simulink model "ADC_Model"  (R2016a)
settings: Solver=ode4  StartTime=t0  StopTime=tf  FixedStep=dt  RelTol=1e-6
InitFcn:
  | sat_model_init
values from neighbouring files (symbols this model uses):
  bias0 = 3/3600*randn(3,1)*pi/180    [sat_model_init.m]
  epoch = [2017 06 01 00 00 00]    [sat_model_init.m]
  gyro_freq = 25    [sat_model_init.m]
  I_max = 1.0    (= 1)    [sat_model_init.m]
  J = [1 ... (first row only)    [sat_model_init.m]
  J_c = [Jx  0  0 ... (first row only)    [sat_model_init.m]
  m = 9    [sat_model_init.m]
  mag_freq = 10    [sat_model_init.m]
  mu = 3.986004415e14    (= 398600441500000)    [sat_model_init.m]
  q0 = [1 ... (first row only)    [sat_model_init.m]
  r0 = (ROT3(omega)*ROT1(inc)*ROT3(Omega))'*[r0*cos(f0) ... (first row only)    [sat_model_init.m]
  Re = 6378.1363e3    (= 6378136.3)    [sat_model_init.m]
  sig_B = 4.5e-8    (= 4.5e-08)    [sat_model_init.m]
  sig_s = 0.1    [sat_model_init.m]
  sig_u = 1*pi/180*1/3600    (= 4.8481368111e-06)    [sat_model_init.m]
  sig_v = (0.0066*pi/180)*2    (= 0.000230383461263)    [sat_model_init.m]
  SP = 4.57e-5    (= 4.57e-05)    [sat_model_init.m]
  sun_freq = 10    [sat_model_init.m]
  v0 = (ROT3(omega)*ROT1(inc)*ROT3(Omega))'*[-mu/h*sin(f0) ... (first row only)    [sat_model_init.m]
  w0 = 0.2*ones(3,1)/sqrt(3)    [sat_model_init.m]
  w_earth = 7.2921158553e-5    (= 7.2921158553e-05)    [sat_model_init.m]
undefined symbols (not defined in the file or in its folder): FACET_model
libraries: vrlib x4
settings Model: Creator=Josue  LastModifiedBy=Graham Voysey
settings DataIOCC: LimitDataPoints=on  SaveFormat=Array  SignalLoggingSaveFormat=ModelDataLogs  SaveState=on
settings OptimizationCC: ExpressionDepthLimit=2147483647  EfficientMapNaN2IntZero=off
settings DebuggingCC: ReadBeforeWriteMsg=DisableAll  WriteAfterWriteMsg=DisableAll  WriteAfterReadMsg=DisableAll  UnderspecifiedInitializationDetection=Classic  MergeDetectMultiDrivingBlocksExec=none  SolverPrmCheckMsg=warning  MultiTaskDSMMsg=warning  MultiTaskCondExecSysMsg=none  FcnCallInpInsideContextMsg=UseLocalSettings  StateNameClashWarn=warning
settings HardwareCC: ProdBitPerPointer=32  ProdLargestAtomicFloat=None  ProdIntDivRoundTo=Undefined  ProdEndianess=Unspecified  ProdWordSize=32  ProdHWDeviceType=32-bit Generic  TargetBitPerPointer=64  TargetLongLongMode=on  TargetIntDivRoundTo=Zero  TargetEndianess=LittleEndian  TargetWordSize=64  TargetHWDeviceType=MATLAB Host  ProdEqTarget=off
settings ModelReferenceCC: PropagateSignalLabelsOutOfModel=off
settings SFSimCC: SimParseCustomCode=off
settings CodeAppCC: MaxIdLength=128
settings GRTTargetCC: CombineOutputUpdateFcns=off  GRTInterface=on
settings ConfigComp: CovModelRefEnable=Off

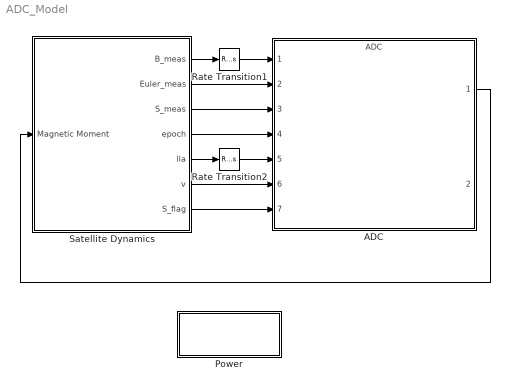
== system ADC_Model ==
  ADC : ModelReference  ModelNameDialog=ADC  SimulationMode=Normal  ModelReferenceVersion=1.1171
  Power : Subsystem
  Rate Transition1 : RateTransition  OutPortSampleTime=.1
  Rate Transition2 : RateTransition  OutPortSampleTime=.1
  Satellite Dynamics : Subsystem
  wires:
  Satellite Dynamics/4(epoch) -> ADC/4
  Satellite Dynamics/1(B_meas) -> Rate Transition1/1
  Satellite Dynamics/2(Euler_meas) -> ADC/2
  Satellite Dynamics/3(S_meas) -> ADC/3
  Satellite Dynamics/5(lla) -> Rate Transition2/1
  Satellite Dynamics/7(S_flag) -> ADC/7
  ADC/1 -> Satellite Dynamics/1(Magnetic Moment)
  Satellite Dynamics/6(v) -> ADC/6
  Rate Transition1/1 -> ADC/1
  Rate Transition2/1 -> ADC/5

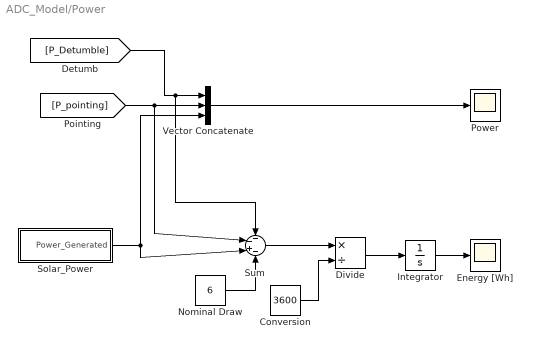
== system ADC_Model/Power ==
  Conversion : Constant  Value=3600
  Divide : Product  Inputs=*/
  Energy [Wh] : Scope
  Integrator : Integrator  InitialCondition=25  LimitOutput=on  UpperSaturationLimit=30  LowerSaturationLimit=0
  Nominal Draw : Constant  Value=6
  Power : Scope
  Solar_Power : Subsystem
  Sum : Sum  Inputs=--+-
  Vector Concatenate : Concatenate  NumInputs=3
  wires:
  [P_Detumble] -> Vector Concatenate/1, Sum/1
  Vector Concatenate/1 -> Power/1
  [P_pointing] -> Sum/2, Vector Concatenate/2
  Solar_Power/1(Power_Generated) -> Vector Concatenate/3, Sum/3
  Nominal Draw/1 -> Sum/4
  Integrator/1 -> Energy [Wh]/1
  Divide/1 -> Integrator/1
  Conversion/1 -> Divide/2
  Sum/1 -> Divide/1

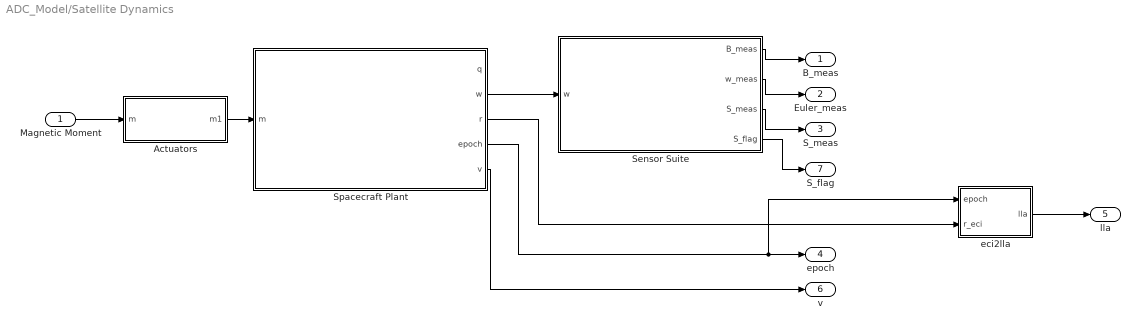
== system ADC_Model/Satellite Dynamics ==
  Magnetic Moment : Inport
  Actuators : Subsystem
  Sensor Suite : Subsystem
  Spacecraft Plant : Subsystem
  eci2lla : MATLAB Function  TreatAsAtomicUnit=on
  B_meas : Outport
  Euler_meas : Outport  Port=2
  S_meas : Outport  Port=3
  epoch : Outport  Port=4
  lla : Outport  Port=5
  v : Outport  Port=6
  S_flag : Outport  Port=7
  wires:
  Spacecraft Plant/2(w) -> Sensor Suite/1(w)
  Magnetic Moment/1 -> Actuators/1(m)
  Sensor Suite/1(B_meas) -> B_meas/1
  Sensor Suite/2(w_meas) -> Euler_meas/1
  Sensor Suite/3(S_meas) -> S_meas/1
  Actuators/1(m1) -> Spacecraft Plant/1(m)
  Spacecraft Plant/5(v) -> v/1
  Spacecraft Plant/4(epoch) -> eci2lla/1(epoch), epoch/1
  Sensor Suite/4(S_flag) -> S_flag/1
  eci2lla/1(lla) -> lla/1
  Spacecraft Plant/3(r) -> eci2lla/2(r_eci)

== system ADC_Model/Power/Solar_Power ==
  Constant2 : Constant  Value=Re
  Constant3 : Constant  Value=FACET_model.Asolar
  Constant6 : Constant  Value=FACET_model.n
  Constant8 : Constant  Value=FACET_model.num_of_faces
  Embedded MATLAB Function : MATLAB Function  TreatAsAtomicUnit=on
  Power_Generated : Outport
  wires:
  Embedded MATLAB Function/1(Power) -> Power_Generated/1
  [R_BtoECI] -> Embedded MATLAB Function/6(R_BtoECI)
  [R_SUN] -> Embedded MATLAB Function/1(R_SUN)
  Constant8/1 -> Embedded MATLAB Function/4(faces)
  [r] -> Embedded MATLAB Function/2(r)
  Constant6/1 -> Embedded MATLAB Function/3(n)
  Constant2/1 -> Embedded MATLAB Function/5(Re)
  Constant3/1 -> Embedded MATLAB Function/7(Pfaces)

== system ADC_Model/Satellite Dynamics/Actuators ==
  m : Inport
  Constant : Constant  Commented=on  Value=0
  I : Constant  Commented=on  Value=I_max
  Interpreted MATLAB Function : MATLABFcn  Commented=on  MATLABFcn=norm
  Power : Scope  Commented=on
  Product : Product  Commented=on  Inputs=3  RndMeth=Zero
  Relational Operator : RelationalOperator  Commented=on  Operator=>  OutDataTypeStr=boolean
  V : Constant  Commented=on  Value=3.3
  dipole : Scope
  m1 : Outport
  wires:
  m/1 -> m1/1, dipole/1, Interpreted MATLAB Function/1
  I/1 -> Product/3
  V/1 -> Product/2
  Product/1 -> Power/1
  Constant/1 -> Relational Operator/2
  Relational Operator/1 -> Product/1
  Interpreted MATLAB Function/1 -> Relational Operator/1

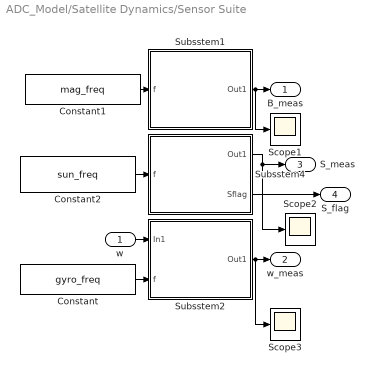
== system ADC_Model/Satellite Dynamics/Sensor Suite ==
  w : Inport
  Constant : Constant  Value=gyro_freq
  Constant1 : Constant  Value=mag_freq
  Constant2 : Constant  Value=sun_freq
  Scope1 : Scope
  Scope2 : Scope
  Scope3 : Scope
  Subsstem1 : Subsystem
      mask Display:
      | fprintf('Magnetometer')
      | port_label('input',1,'f')
  Subsstem2 : Subsystem
      mask Display:
      | fprintf('Gyro')
      | port_label('input',1,'w')
      | port_label('input',2,'f')
  Subsstem4 : Subsystem
      mask Display:
      | fprintf('Sun Sensor')
      | port_label('input',1,'f')
  B_meas : Outport
  w_meas : Outport  Port=2
  S_meas : Outport  Port=3
  S_flag : Outport  Port=4
  wires:
  Constant1/1 -> Subsstem1/1(f)
  Subsstem1/1(Out1) -> Scope1/1, B_meas/1
  w/1 -> Subsstem2/1(In1)
  Constant/1 -> Subsstem2/2(f)
  Subsstem2/1(Out1) -> Scope3/1, w_meas/1
  Constant2/1 -> Subsstem4/1(f)
  Subsstem4/1(Out1) -> Scope2/1, S_meas/1
  Subsstem4/2(Sflag) -> S_flag/1

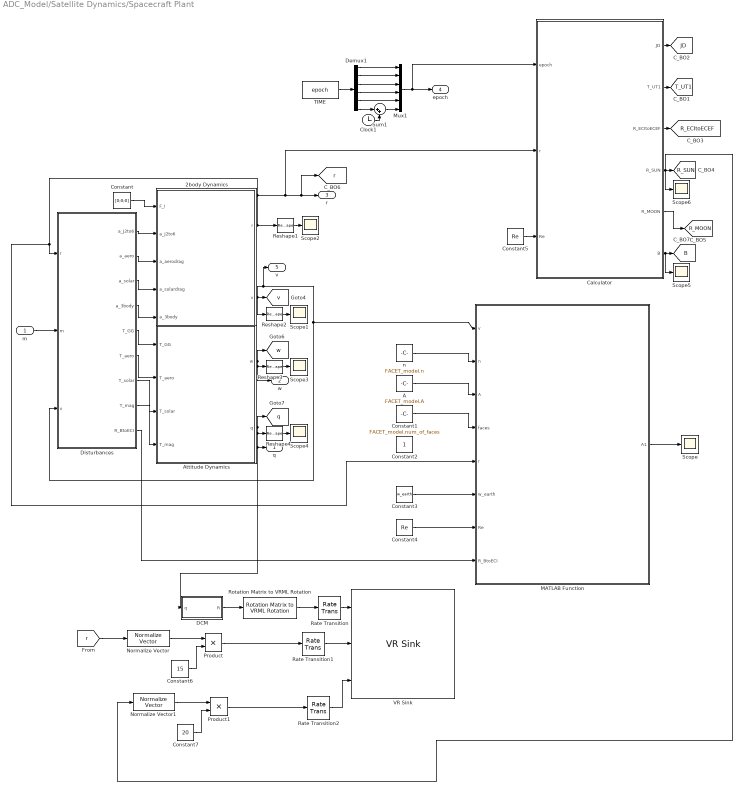
== system ADC_Model/Satellite Dynamics/Spacecraft Plant ==
  m : Inport
  2body Dynamics : Subsystem
  A : Constant  Value=FACET_model.A
  Attitude Dynamics : Subsystem
  Calculator : MATLAB Function  TreatAsAtomicUnit=on
  Clock1 : Clock
  Constant : Constant  Value=[0;0;0]
  Constant1 : Constant  Value=FACET_model.num_of_faces
  Constant2 : Constant
  Constant3 : Constant  Value=w_earth
  Constant4 : Constant  Value=Re
  Constant5 : Constant  Value=Re
  Constant6 : Constant  Value=15
  Constant7 : Constant  Value=20
  DCM : MATLAB Function  TreatAsAtomicUnit=on
  Demux1 : Demux  Outputs=6
  Disturbances : Subsystem
  MATLAB Function : MATLAB Function  TreatAsAtomicUnit=on
  Mux1 : Mux  Inputs=6
  Normalize Vector : vrlib/Utilities/Normalize Vector  maxzero=0
  Normalize Vector1 : vrlib/Utilities/Normalize Vector  maxzero=0
  Product : Product
  Product1 : Product
  Rate Transition : RateTransition  OutPortSampleTime=1
  Rate Transition1 : RateTransition  OutPortSampleTime=1
  Rate Transition2 : RateTransition  OutPortSampleTime=1
  Reshape{1..4} (4 alike) : Reshape
  Rotation Matrix to VRML Rotation : vrlib/Utilities/Rotation Matrix to VRML Rotation  maxzero=1e-12
  Scope{,1..6} (7 alike) : Scope
  Sum1 : Sum  Inputs=|++
  TIME : Constant  Value=epoch
  VR Sink : vrlib/VR Sink  InstantiateOnLoad=on  SampleTime=1  ViewEnable=on  RemoteChange=off  RemoteView=off  FieldsWritten=ANDESITE.rotation.4.1.1.double#ANDESITE.translation.3.1.1.double#Sun.translation.3.1.1.double  WorldFileName=ANDESITE_attitude.wrl  AutoView=on  VideoDimensions=[]  AllowVariableSize=off
  n : Constant  Value=FACET_model.n
  q : Outport
  w : Outport  Port=2
  r : Outport  Port=3
  epoch : Outport  Port=4
  v : Outport  Port=5
  tag scope: B=global, JD=global, R_ECItoECEF=global, R_MOON=global, R_SUN=global, T_UT1=global, q=global, r=global, v=global, w=global
  wires:
  Reshape3/1 -> Scope3/1
  Reshape2/1 -> Scope1/1
  Reshape1/1 -> Scope2/1
  Reshape4/1 -> Scope4/1
  2body Dynamics/2(v) -> [v], Reshape2/1, v/1, Disturbances/3(v), MATLAB Function/1(v)
  Disturbances/1(a_J2to6) -> 2body Dynamics/2(a_J2to6)
  Disturbances/2(a_aero) -> 2body Dynamics/3(a_aerodrag)
  Disturbances/3(a_solar) -> 2body Dynamics/4(a_solardrag)
  Disturbances/4(a_3body) -> 2body Dynamics/5(a_3body)
  Disturbances/5(T_GG) -> Attitude Dynamics/1(T_GG)
  Disturbances/6(T_aero) -> Attitude Dynamics/2(T_aero)
  Disturbances/7(T_solar) -> Attitude Dynamics/3(T_solar)
  Disturbances/8(T_mag) -> Attitude Dynamics/4(T_mag)
  m/1 -> Disturbances/2(m)
  Attitude Dynamics/2(q) -> DCM/1(q), q/1, Reshape4/1, [q]
  Attitude Dynamics/1(w) -> Reshape3/1, w/1, [w]
  Constant/1 -> 2body Dynamics/1(F_I)
  n/1 -> MATLAB Function/2(n)
  A/1 -> MATLAB Function/3(A)
  Constant1/1 -> MATLAB Function/4(faces)
  Constant4/1 -> MATLAB Function/7(Re)
  Constant3/1 -> MATLAB Function/6(w_earth)
  Disturbances/9(R_BtoECI) -> MATLAB Function/8(R_BtoECI)
  MATLAB Function/1(A1) -> Scope/1
  Demux1/2 -> Mux1/2
  Demux1/1 -> Mux1/1
  Demux1/5 -> Mux1/5
  Demux1/4 -> Mux1/4
  Demux1/3 -> Mux1/3
  Sum1/1 -> Mux1/6
  Demux1/6 -> Sum1/1
  TIME/1 -> Demux1/1
  Clock1/1 -> Sum1/2
  Calculator/1(JD) -> [JD]
  Calculator/2(T_UT1) -> [T_UT1]
  Calculator/3(R_ECItoECEF) -> [R_ECItoECEF]
  Calculator/4(R_SUN) -> Scope6/1, Normalize Vector1/1, [R_SUN]
  Calculator/5(R_MOON) -> [R_MOON]
  Calculator/6(B) -> [B], Scope5/1
  Mux1/1 -> Calculator/1(epoch), epoch/1
  Constant5/1 -> Calculator/3(Re)
  2body Dynamics/1(r) -> [r], r/1, Calculator/2(r), Disturbances/1(r), MATLAB Function/5(r), Reshape1/1
  DCM/1(R) -> Rotation Matrix to VRML Rotation/1
  Rotation Matrix to VRML Rotation/1 -> Rate Transition/1
  Constant6/1 -> Product/2
  Normalize Vector/1 -> Product/1
  Product/1 -> Rate Transition1/1
  [r] -> Normalize Vector/1
  Rate Transition/1 -> VR Sink/1
  Rate Transition1/1 -> VR Sink/2
  Constant7/1 -> Product1/2
  Normalize Vector1/1 -> Product1/1
  Product1/1 -> Rate Transition2/1
  Rate Transition2/1 -> VR Sink/3

== system ADC_Model/Satellite Dynamics/Sensor Suite/Subsstem1 ==
  f : Inport
  Clock : Clock
  Constant1 : Constant  Value=sig_B
  Embedded MATLAB Function : MATLAB Function  TreatAsAtomicUnit=on
  Memory : Memory  X0=[0;0;0]
  Out1 : Outport
  wires:
  Embedded MATLAB Function/1(B_meas) -> Out1/1, Memory/1
  Memory/1 -> Embedded MATLAB Function/6(B_hold)
  f/1 -> Embedded MATLAB Function/3(f)
  [B] -> Embedded MATLAB Function/1(B)
  [R_BtoECI] -> Embedded MATLAB Function/5(R_BtoECI)
  Constant1/1 -> Embedded MATLAB Function/4(sig_B)
  Clock/1 -> Embedded MATLAB Function/2(t)

== system ADC_Model/Satellite Dynamics/Sensor Suite/Subsstem2 ==
  In1 : Inport
  f : Inport  Port=2
  Clock : Clock
  Constant : Constant  Value=sig_u
  Constant1 : Constant  Value=sig_v
  Embedded MATLAB Function : MATLAB Function  TreatAsAtomicUnit=on
  Integrator : Integrator  InitialCondition=bias0
  Memory : Memory  X0=w0
  Out1 : Outport
  wires:
  Clock/1 -> Embedded MATLAB Function/5(t)
  Memory/1 -> Embedded MATLAB Function/7(w_hold)
  In1/1 -> Embedded MATLAB Function/1(w)
  f/1 -> Embedded MATLAB Function/6(f)
  Embedded MATLAB Function/2(w_meas) -> Out1/1, Memory/1
  Embedded MATLAB Function/1(bias_dot) -> Integrator/1
  Integrator/1 -> Embedded MATLAB Function/2(bias)
  Constant/1 -> Embedded MATLAB Function/3(sig_u)
  Constant1/1 -> Embedded MATLAB Function/4(sig_v)

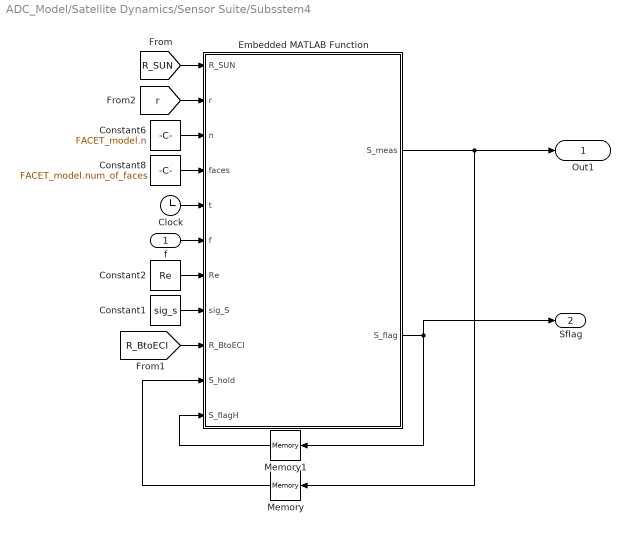
== system ADC_Model/Satellite Dynamics/Sensor Suite/Subsstem4 ==
  f : Inport
  Clock : Clock
  Constant1 : Constant  Value=sig_s
  Constant2 : Constant  Value=Re
  Constant6 : Constant  Value=FACET_model.n
  Constant8 : Constant  Value=FACET_model.num_of_faces
  Embedded MATLAB Function : MATLAB Function  TreatAsAtomicUnit=on
  Memory : Memory  X0=[0;0;0]
  Memory1 : Memory
  Out1 : Outport
  Sflag : Outport  Port=2
  wires:
  Clock/1 -> Embedded MATLAB Function/5(t)
  Constant1/1 -> Embedded MATLAB Function/8(sig_S)
  [R_BtoECI] -> Embedded MATLAB Function/9(R_BtoECI)
  [R_SUN] -> Embedded MATLAB Function/1(R_SUN)
  f/1 -> Embedded MATLAB Function/6(f)
  Memory/1 -> Embedded MATLAB Function/10(S_hold)
  Constant6/1 -> Embedded MATLAB Function/3(n)
  [r] -> Embedded MATLAB Function/2(r)
  Constant8/1 -> Embedded MATLAB Function/4(faces)
  Constant2/1 -> Embedded MATLAB Function/7(Re)
  Embedded MATLAB Function/1(S_meas) -> Memory/1, Out1/1
  Embedded MATLAB Function/2(S_flag) -> Sflag/1, Memory1/1
  Memory1/1 -> Embedded MATLAB Function/11(S_flagH)

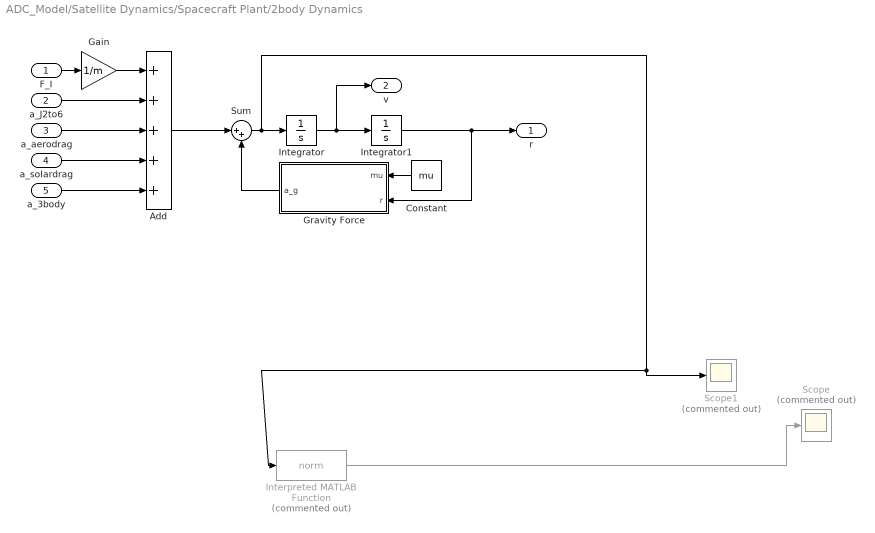
== system ADC_Model/Satellite Dynamics/Spacecraft Plant/2body Dynamics ==
  F_I : Inport
  a_J2to6 : Inport  Port=2
  a_aerodrag : Inport  Port=3
  a_solardrag : Inport  Port=4
  a_3body : Inport  Port=5
  Add : Sum  Inputs=+++++
  Constant : Constant  Value=mu
  Gain : Gain  Gain=1/m
  Gravity Force : MATLAB Function  TreatAsAtomicUnit=on
  Integrator : Integrator  InitialCondition=v0
  Integrator1 : Integrator  InitialCondition=r0
  Interpreted MATLAB Function : MATLABFcn  Commented=on  MATLABFcn=norm
  Scope : Scope  Commented=on
  Scope1 : Scope  Commented=on
  Sum : Sum  Inputs=|++
  r : Outport
  v : Outport  Port=2
  wires:
  Add/1 -> Sum/1
  Gain/1 -> Add/1
  a_3body/1 -> Add/5
  a_solardrag/1 -> Add/4
  a_aerodrag/1 -> Add/3
  a_J2to6/1 -> Add/2
  Constant/1 -> Gravity Force/1(mu)
  Integrator1/1 -> r/1, Gravity Force/2(r)
  Integrator/1 -> v/1, Integrator1/1
  Gravity Force/1(a_g) -> Sum/2
  Sum/1 -> Integrator/1, Scope1/1, Interpreted MATLAB Function/1
  F_I/1 -> Gain/1
  Interpreted MATLAB Function/1 -> Scope/1

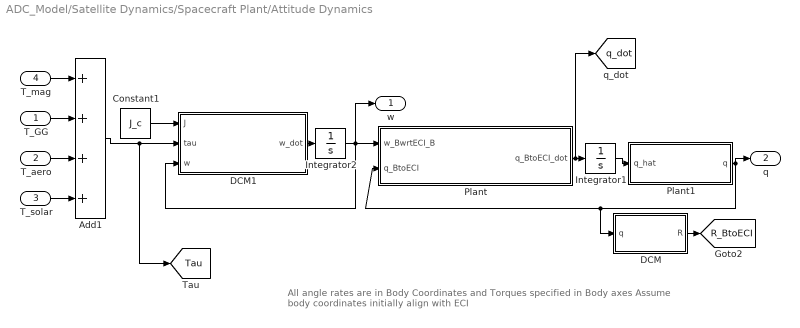
== system ADC_Model/Satellite Dynamics/Spacecraft Plant/Attitude Dynamics ==
  note: All angle rates are in Body Coordinates and Torques specified in Body axes
      | Assume body coordinates initially align with ECI
  T_GG : Inport
  T_aero : Inport  Port=2
  T_solar : Inport  Port=3
  T_mag : Inport  Port=4
  Add1 : Sum  Inputs=++++
  Constant1 : Constant  Value=J_c
  DCM : MATLAB Function  TreatAsAtomicUnit=on
  DCM1 : MATLAB Function  TreatAsAtomicUnit=on
  Integrator1 : Integrator  InitialCondition=q0
  Integrator2 : Integrator  InitialCondition=w0
  Plant : MATLAB Function  TreatAsAtomicUnit=on
  Plant1 : MATLAB Function  TreatAsAtomicUnit=on
  w : Outport
  q : Outport  Port=2
  tag scope: R_BtoECI=global, Tau=global, q_dot=global
  wires:
  Integrator1/1 -> Plant1/1(q_hat)
  T_solar/1 -> Add1/4
  T_aero/1 -> Add1/3
  T_GG/1 -> Add1/2
  Plant1/1(q) -> q/1, Plant/2(q_BtoECI), DCM/1(q)
  DCM1/1(w_dot) -> Integrator2/1
  Add1/1 -> [Tau], DCM1/2(tau)
  Constant1/1 -> DCM1/1(J)
  Plant/1(q_BtoECI_dot) -> [q_dot], Integrator1/1
  Integrator2/1 -> Plant/1(w_BwrtECI_B), w/1, DCM1/3(w)
  DCM/1(R) -> [R_BtoECI]
  T_mag/1 -> Add1/1

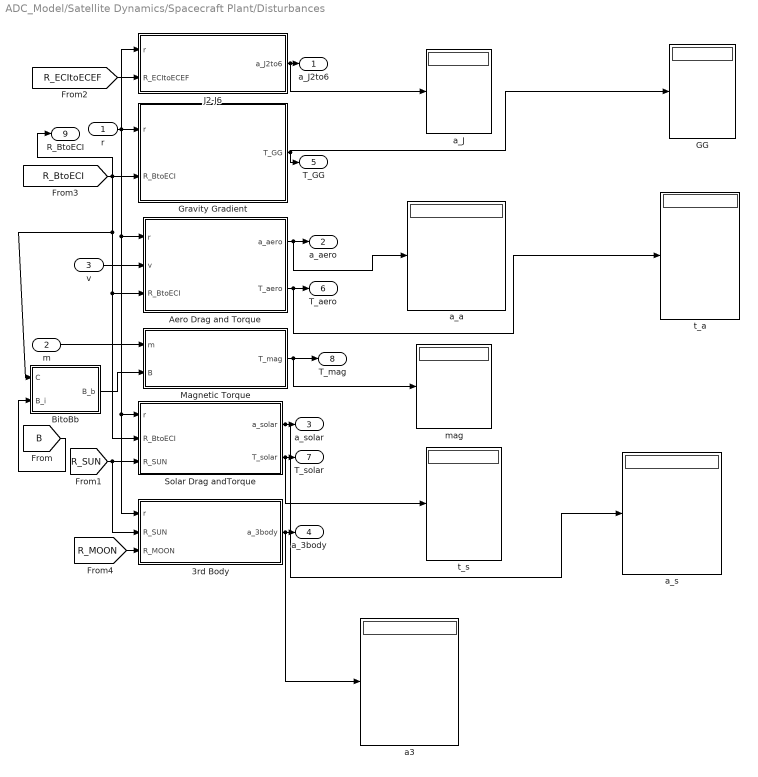
== system ADC_Model/Satellite Dynamics/Spacecraft Plant/Disturbances ==
  r : Inport
  m : Inport  Port=2
  v : Inport  Port=3
  3rd Body : Subsystem  TreatAsAtomicUnit=on
  Aero Drag and Torque : Subsystem  TreatAsAtomicUnit=on
  BitoBb : MATLAB Function  TreatAsAtomicUnit=on
  GG : Display
  Gravity Gradient : Subsystem  TreatAsAtomicUnit=on
  J2-J6 : Subsystem  TreatAsAtomicUnit=on
  Magnetic Torque : Subsystem  TreatAsAtomicUnit=on
  Solar Drag andTorque : Subsystem  TreatAsAtomicUnit=on
  a3 : Display
  a_J : Display
  a_a : Display
  a_s : Display
  mag : Display
  t_a : Display
  t_s : Display
  a_J2to6 : Outport
  a_aero : Outport  Port=2
  a_solar : Outport  Port=3
  a_3body : Outport  Port=4
  T_GG : Outport  Port=5
  T_aero : Outport  Port=6
  T_solar : Outport  Port=7
  T_mag : Outport  Port=8
  R_BtoECI : Outport  Port=9
  wires:
  v/1 -> Aero Drag and Torque/2(v)
  [R_BtoECI] -> Gravity Gradient/2(R_BtoECI), Solar Drag andTorque/2(R_BtoECI), Aero Drag and Torque/3(R_BtoECI), BitoBb/1(C), R_BtoECI/1
  r/1 -> Aero Drag and Torque/1(r), Solar Drag andTorque/1(r), 3rd Body/1(r), Gravity Gradient/1(r), J2-J6/1(r)
  Aero Drag and Torque/1(a_aero) -> a_a/1, a_aero/1
  Solar Drag andTorque/1(a_solar) -> a_s/1, a_solar/1
  [R_ECItoECEF] -> J2-J6/2(R_ECItoECEF)
  [R_SUN] -> Solar Drag andTorque/3(R_SUN), 3rd Body/2(R_SUN)
  [R_MOON] -> 3rd Body/3(R_MOON)
  m/1 -> Magnetic Torque/1(m)
  BitoBb/1(B_b) -> Magnetic Torque/2(B)
  [B] -> BitoBb/2(B_i)
  J2-J6/1(a_J2to6) -> a_J/1, a_J2to6/1
  Gravity Gradient/1(T_GG) -> T_GG/1, GG/1
  Aero Drag and Torque/2(T_aero) -> t_a/1, T_aero/1
  3rd Body/1(a_3body) -> a3/1, a_3body/1
  Solar Drag andTorque/2(T_solar) -> t_s/1, T_solar/1
  Magnetic Torque/1(T_mag) -> mag/1, T_mag/1

== system ADC_Model/Satellite Dynamics/Spacecraft Plant/Disturbances/3rd Body ==
  r : Inport
  R_SUN : Inport  Port=2
  R_MOON : Inport  Port=3
  Third Body Effects : MATLAB Function  TreatAsAtomicUnit=on
  a_3body : Outport
  wires:
  Third Body Effects/1(a_3body) -> a_3body/1
  R_SUN/1 -> Third Body Effects/2(R_SUN)
  r/1 -> Third Body Effects/1(r)
  R_MOON/1 -> Third Body Effects/3(R_MOON)

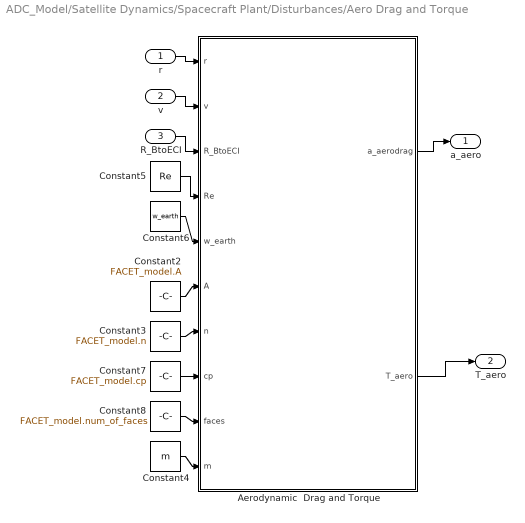
== system ADC_Model/Satellite Dynamics/Spacecraft Plant/Disturbances/Aero Drag and Torque ==
  r : Inport
  v : Inport  Port=2
  R_BtoECI : Inport  Port=3
  Aerodynamic  Drag and Torque : MATLAB Function  TreatAsAtomicUnit=on
  Constant2 : Constant  Value=FACET_model.A
  Constant3 : Constant  Value=FACET_model.n
  Constant4 : Constant  Value=m
  Constant5 : Constant  Value=Re
  Constant6 : Constant  Value=w_earth
  Constant7 : Constant  Value=FACET_model.cp
  Constant8 : Constant  Value=FACET_model.num_of_faces
  a_aero : Outport
  T_aero : Outport  Port=2
  wires:
  Aerodynamic  Drag and Torque/2(T_aero) -> T_aero/1
  R_BtoECI/1 -> Aerodynamic  Drag and Torque/3(R_BtoECI)
  v/1 -> Aerodynamic  Drag and Torque/2(v)
  r/1 -> Aerodynamic  Drag and Torque/1(r)
  Aerodynamic  Drag and Torque/1(a_aerodrag) -> a_aero/1
  Constant4/1 -> Aerodynamic  Drag and Torque/10(m)
  Constant5/1 -> Aerodynamic  Drag and Torque/4(Re)
  Constant6/1 -> Aerodynamic  Drag and Torque/5(w_earth)
  Constant2/1 -> Aerodynamic  Drag and Torque/6(A)
  Constant3/1 -> Aerodynamic  Drag and Torque/7(n)
  Constant7/1 -> Aerodynamic  Drag and Torque/8(cp)
  Constant8/1 -> Aerodynamic  Drag and Torque/9(faces)

== system ADC_Model/Satellite Dynamics/Spacecraft Plant/Disturbances/Gravity Gradient ==
  r : Inport
  R_BtoECI : Inport  Port=2
  Constant : Constant  Value=mu
  Constant1 : Constant  Value=J_c
  Gravity Gradient : MATLAB Function  TreatAsAtomicUnit=on
  T_GG : Outport
  wires:
  Gravity Gradient/1(T_GG) -> T_GG/1
  r/1 -> Gravity Gradient/1(r)
  R_BtoECI/1 -> Gravity Gradient/2(R_BtoECI)
  Constant1/1 -> Gravity Gradient/3(J_c)
  Constant/1 -> Gravity Gradient/4(mu)

== system ADC_Model/Satellite Dynamics/Spacecraft Plant/Disturbances/J2-J6 ==
  r : Inport
  R_ECItoECEF : Inport  Port=2
  Constant : Constant  Value=mu
  Constant1 : Constant  Value=Re
  Constant2 : Constant  Value=J
  J2-J6 Effect : MATLAB Function  TreatAsAtomicUnit=on
  a_J2to6 : Outport
  wires:
  J2-J6 Effect/1(a_J2to6) -> a_J2to6/1
  r/1 -> J2-J6 Effect/1(r_ECI)
  Constant/1 -> J2-J6 Effect/3(mu)
  R_ECItoECEF/1 -> J2-J6 Effect/2(R_ECItoECEF)
  Constant1/1 -> J2-J6 Effect/4(Re)
  Constant2/1 -> J2-J6 Effect/5(J)

== system ADC_Model/Satellite Dynamics/Spacecraft Plant/Disturbances/Magnetic Torque ==
  m : Inport
  B : Inport  Port=2
  Cross Product : Subsystem
      mask Display: plot([.05 .95],[.05 .95],[.05 .95],[.95 .05])
  MATLAB Function : MATLAB Function  Commented=on  TreatAsAtomicUnit=on
  T_mag : Outport
  wires:
  m/1 -> Cross Product/1(In1)
  Cross Product/1(Out1) -> T_mag/1
  B/1 -> Cross Product/2(In2)

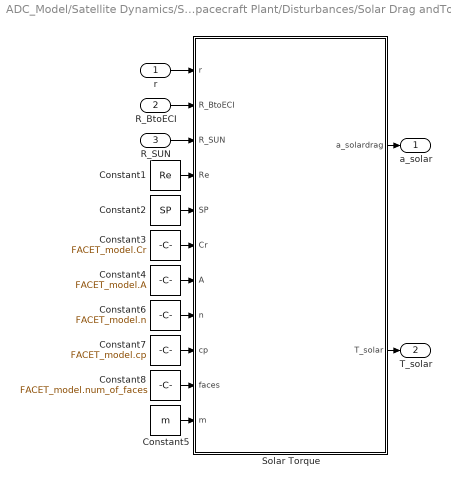
== system ADC_Model/Satellite Dynamics/Spacecraft Plant/Disturbances/Solar Drag andTorque ==
  r : Inport
  R_BtoECI : Inport  Port=2
  R_SUN : Inport  Port=3
  Constant1 : Constant  Value=Re
  Constant2 : Constant  Value=SP
  Constant3 : Constant  Value=FACET_model.Cr
  Constant4 : Constant  Value=FACET_model.A
  Constant5 : Constant  Value=m
  Constant6 : Constant  Value=FACET_model.n
  Constant7 : Constant  Value=FACET_model.cp
  Constant8 : Constant  Value=FACET_model.num_of_faces
  Solar Torque : MATLAB Function  TreatAsAtomicUnit=on
  a_solar : Outport
  T_solar : Outport  Port=2
  wires:
  R_BtoECI/1 -> Solar Torque/2(R_BtoECI)
  r/1 -> Solar Torque/1(r)
  Solar Torque/2(T_solar) -> T_solar/1
  Solar Torque/1(a_solardrag) -> a_solar/1
  R_SUN/1 -> Solar Torque/3(R_SUN)
  Constant1/1 -> Solar Torque/4(Re)
  Constant2/1 -> Solar Torque/5(SP)
  Constant5/1 -> Solar Torque/11(m)
  Constant3/1 -> Solar Torque/6(Cr)
  Constant4/1 -> Solar Torque/7(A)
  Constant6/1 -> Solar Torque/8(n)
  Constant7/1 -> Solar Torque/9(cp)
  Constant8/1 -> Solar Torque/10(faces)

== system ADC_Model/Satellite Dynamics/Spacecraft Plant/Disturbances/Magnetic Torque/Cross Product ==
  In1 : Inport
  In2 : Inport  Port=2
  Assemble Matrix : Subsystem
  Constant : Constant  Value=0
  Demux : Demux  Outputs=3
  Product : Product  Multiplication=Matrix(*)  RndMeth=Zero
  Unary Minus : UnaryMinus
  Unary Minus1 : UnaryMinus
  Unary Minus2 : UnaryMinus
  Out1 : Outport
  wires:
  In1/1 -> Demux/1
  Constant/1 -> Assemble Matrix/1(A11), Assemble Matrix/5(A22), Assemble Matrix/9(A33)
  Unary Minus/1 -> Assemble Matrix/2(A12)
  Demux/3 -> Unary Minus/1, Assemble Matrix/4(A21)
  Demux/2 -> Assemble Matrix/3(A13), Unary Minus2/1
  Demux/1 -> Unary Minus1/1, Assemble Matrix/8(A32)
  Unary Minus1/1 -> Assemble Matrix/6(A23)
  Unary Minus2/1 -> Assemble Matrix/7(A31)
  Assemble Matrix/1(A) -> Product/1
  In2/1 -> Product/2
  Product/1 -> Out1/1

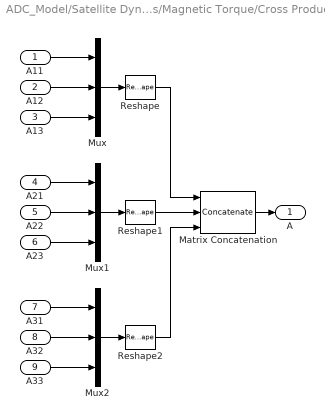
== system ADC_Model/Satellite Dynamics/Spacecraft Plant/Disturbances/Magnetic Torque/Cross Product/Assemble Matrix ==
  A11 : Inport
  A12 : Inport  Port=2
  A13 : Inport  Port=3
  A21 : Inport  Port=4
  A22 : Inport  Port=5
  A23 : Inport  Port=6
  A31 : Inport  Port=7
  A32 : Inport  Port=8
  A33 : Inport  Port=9
  Matrix Concatenation : Concatenate  NumInputs=3  Mode=Multidimensional array
  Mux : Mux  Inputs=3
  Mux1 : Mux  Inputs=3
  Mux2 : Mux  Inputs=3
  Reshape : Reshape  OutputDimensionality=Row vector (2-D)
  Reshape1 : Reshape  OutputDimensionality=Row vector (2-D)
  Reshape2 : Reshape  OutputDimensionality=Row vector (2-D)
  A : Outport
  wires:
  A11/1 -> Mux/1
  A12/1 -> Mux/2
  A13/1 -> Mux/3
  A21/1 -> Mux1/1
  A22/1 -> Mux1/2
  A23/1 -> Mux1/3
  A31/1 -> Mux2/1
  A32/1 -> Mux2/2
  A33/1 -> Mux2/3
  Mux/1 -> Reshape/1
  Mux1/1 -> Reshape1/1
  Mux2/1 -> Reshape2/1
  Reshape1/1 -> Matrix Concatenation/2
  Reshape/1 -> Matrix Concatenation/1
  Reshape2/1 -> Matrix Concatenation/3
  Matrix Concatenation/1 -> A/1

== matlab function ADC_Model/Satellite Dynamics/Spacecraft Plant/2body Dynamics/Gravity Force ==
  data: mu input; a_g output; r input
function a_g = twobody(mu,r)

a_g = -(mu/norm(r)^3)*r;

== matlab function ADC_Model/Satellite Dynamics/Spacecraft Plant/Attitude Dynamics/Plant1 ==
  data: q_hat input; q output
function q = q_norm(q_hat)
% This block supports an embeddable subset of the MATLAB language.
% See the help menu for details. 

q = q_hat/norm(q_hat);

end

== matlab function ADC_Model/Satellite Dynamics/Spacecraft Plant/Attitude Dynamics/DCM1 ==
  data: J input; w_dot output; tau input; w input
function w_dot = Euler(J,tau,w)

w_dot = J\(tau-skew(w)*J*w);

end

function A = skew(x)

A = [0    -x(3)  x(2);
     x(3)  0    -x(1);
    -x(2)  x(1)  0];
 
end

== matlab function ADC_Model/Satellite Dynamics/Spacecraft Plant/Attitude Dynamics/DCM ==
  data: q input; R output
function R = DCM(q)

R = Psi_matrix(q)'*Xi_matrix(q);

end

function A = Xi_matrix(q)
A = [q(4)*eye(3)+skew(q(1:3));
    -q(1:3)'];
end

function A = Psi_matrix(q)
A = [q(4)*eye(3)-skew(q(1:3));
    -q(1:3)'];
end

function A = skew(x)
A = [0 -x(3) x(2);
     x(3) 0  -x(1);
    -x(2) x(1) 0];
end

== matlab function ADC_Model/Satellite Dynamics/Sensor Suite/Subsstem1/Embedded MATLAB Function ==
  data: B_meas output; B input; t input; f input; sig_B input; R_BtoECI input; B_hold input
function B_meas = Magnetometer(B,t,f,sig_B,R_BtoECI,B_hold)

if mod(t,1/f) == 0
    B_meas = R_BtoECI'*(B + sig_B*norm(B)*randn(3,1));
%     B_meas = R_BtoECI'*B;
   
else
    B_meas = B_hold;
end

end

== matlab function ADC_Model/Satellite Dynamics/Sensor Suite/Subsstem2/Embedded MATLAB Function ==
  data: bias_dot output; w input; bias input; sig_u input; sig_v input; t input; f input; w_meas output; w_hold input
function [bias_dot,w_meas] = Gyro(w,bias,sig_u,sig_v,t,f,w_hold)

if mod(t,1/f) == 0
    w_meas = w + sig_v*randn(3,1) + bias;
else
    w_meas = w_hold;
end

bias_dot = sig_u*randn(3,1);

end

== matlab function ADC_Model/Satellite Dynamics/eci2lla ==
  data: epoch input; lla output; r_eci input
% USAGE:
% [lat,lon,alt] = ecef2lla(epoch,r_eci)
%
% lat = geodetic latitude (radians)
% lon = longitude (radians)
% alt = height above WGS84 ellipsoid (m)
% x = ECEF X-coordinate (m)
% y = ECEF Y-coordinate (m)
% z = ECEF Z-coordinate (m)
%
% Notes: (1) This function assumes the WGS84 model.
%        (2) Latitude is customary geodetic (not geocentric).
%        (3) Inputs may be scalars, vectors, or matrices of the same
%            size and shape. Outputs will have that same size and shape.

function lla  = eci2lla(epoch,r_eci)


Re = 6378.1363e3;
%Compute the Julian Date (JD) from a Gregorian Date (UT1) input
yr=epoch(1);  %(year)
mo=epoch(2);  %(month)
d=epoch(3);  %(day)
h=epoch(4);  %(hr)
min=epoch(5);  %(min)
s=epoch(6);  %(sec)
JD=367*yr-floor(7/4*(yr+floor((mo+9)/12)))+floor(275*mo/9)+d+1721013.5+(((s/60+min)/60)+h)/24;  %(JD)

%Compute the Universal Time (UT) from JD
T_UT1 = (JD-2451545.0)/36525;

%Compute the Greenwich Mean Sidereal Time (GMST) from UT
GMST = 67310.54841 + (876600.0*3600.0 + 8640184.812866)*T_UT1 + 0.093104*T_UT1^2 - 6.2E-6*T_UT1^3;
G0 = rem(GMST,86400)/240;
if G0 < 0
    G0 = -(-G0-360);
end
%truncate GMST between 0 and 2pi
GMST = G0*pi/180;  %(rad)

%Compute the Direction Cosine Matrix (DCM) for converting vectors in 
%Earth-Centered Inertial (ECI) frame to vectors in Earth-Centered 
%Earth-Fixed (ECEF) frame
R_ECItoECEF = ROT3(GMST);

r_ecf = R_ECItoECEF*r_eci;

x=r_ecf(1);
y=r_ecf(2);
z=r_ecf(3);

% WGS84 ellipsoid constants:
a = 6378137;
e = 8.1819190842622e-2;

% calculations: make sure angles are right
b   = sqrt(a^2*(1-e^2));
ep  = sqrt((a^2-b^2)/b^2);
p   = sqrt(x.^2+y.^2);
th  = atan2(a*z,b*p);
lon = atan2d(y,x);
lat = atan2d((z+ep^2.*b.*sin(th).^3),(p-e^2.*a.*cos(th).^3));
N   = a./sqrt(1-e^2.*sind(lat).^2);
alt = p./cosd(lat)-N;

% return lon in range [0,2*pi)
lon = mod(lon,360);

% correct for numerical instability in altitude near exact poles:
% (after this correction, error is about 2 millimeters, which is about
% the same as the numerical precision of the overall function)

k=abs(x)<1 & abs(y)<1;
alt(k) = abs(z(k))-b;

lla=[lat,lon,alt];
return

== matlab function ADC_Model/Satellite Dynamics/Sensor Suite/Subsstem4/Embedded MATLAB Function ==
  data: S_meas output; R_SUN input; r input; n input; faces input; t input; f input; Re input; sig_S input; R_BtoECI input; S_hold input; S_flagH input; S_flag output
function [S_meas, S_flag]  = Sun_Sensor(R_SUN,r,n,faces,t,f,Re,sig_S,R_BtoECI,S_hold,S_flagH)

if mod(t,1/f) == 0
    r_sun = -R_BtoECI'*(r - R_SUN);

    S_meas = [0;0;0];
    S_flag = 1;
    
    temp1 = dot(r/Re,R_SUN/Re);
    r1 = norm(r/Re);
    r2 = norm(R_SUN/Re);
    tau_min = (r1^2 - temp1)/(r1^2 + r2^2 - 2*temp1);

    LOS = (tau_min < 0) + (tau_min > 1);
    other = (1-tau_min)*r1^2 + temp1*tau_min;
    LOS = LOS + (other >= 1);
    
    if LOS
        for i = 1:faces
            cos_alf = dot(r_sun/norm(r_sun),n(1:3,i));
            if cos_alf > 0
                S_meas = S_meas + (cos_alf + sig_S*(1-cos_alf)*randn(1))*n(1:3,i);
            end
        end
        S_meas = S_meas/norm(S_meas);
    else
        S_meas = S_hold;
        S_flag = 0;
    end
else
    S_meas = S_hold;
    S_flag = S_flagH;
end

end

== matlab function ADC_Model/Satellite Dynamics/Spacecraft Plant/Disturbances/BitoBb ==
  data: C input; B_b output; B_i input
function B_b = BitoBb(C,B_i)
%#codegen

B_b=C'*B_i;

== matlab function ADC_Model/Satellite Dynamics/Spacecraft Plant/Calculator ==
  data: epoch input; r input; JD output; T_UT1 output; R_ECItoECEF output; R_SUN output; R_MOON output; B output; Re input
function [JD,T_UT1,R_ECItoECEF,R_SUN,R_MOON,B] =space_env(epoch,r,Re)

%Compute the Julian Date (JD) from a Gregorian Date (UT1) input
yr=epoch(1);  %(year)
mo=epoch(2);  %(month)
d=epoch(3);  %(day)
h=epoch(4);  %(hr)
min=epoch(5);  %(min)
s=epoch(6);  %(sec)
JD=367*yr-floor(7/4*(yr+floor((mo+9)/12)))+floor(275*mo/9)+d+1721013.5+(((s/60+min)/60)+h)/24;  %(JD)

%Compute the Universal Time (UT) from JD
T_UT1 = (JD-2451545.0)/36525;

%Compute the Greenwich Mean Sidereal Time (GMST) from UT
GMST = 67310.54841 + (876600.0*3600.0 + 8640184.812866)*T_UT1 + 0.093104*T_UT1^2 - 6.2E-6*T_UT1^3;
G0 = rem(GMST,86400)/240;
if G0 < 0
    G0 = -(-G0-360);
end
%truncate GMST between 0 and 2pi
GMST = G0*pi/180;  %(rad)

%Compute the Direction Cosine Matrix (DCM) for converting vectors in 
%Earth-Centered Inertial (ECI) frame to vectors in Earth-Centered 
%Earth-Fixed (ECEF) frame
R_ECItoECEF = ROT3(GMST);

%Compute the Sun vector based on the UT
R_SUN = r_sun(T_UT1);

%Compute the Moon vector based on the UT
R_MOON = r_moon(T_UT1,Re);

%Compute the Earth's magnetic vector in the ECI frame
B = Dipole_model(r,GMST,Re);  %(T)

end

function A = ROT3(theta)

A = [cos(theta) sin(theta) 0;
    -sin(theta) cos(theta) 0;
     0          0          1];
 
end

function r = r_sun(T_UT1)

lambdaM = 280.4606184+36000.77005361*T_UT1;  %(°)
M = (357.5277233+35999.05034*T_UT1)*pi/180.0;  %(rad)
lambdaecliptic = (lambdaM+1.914666471*sin(M)+0.019994643*sin(2*M))*pi/180.0;  %(rad)
E = (23.439291-0.0130042*T_UT1)*pi/180.0;  %(rad)
Rs = (1.000140612-0.016708617*cos(M)-0.000139589*cos(2*M))*149598000*10^3;  %(m)
r = Rs*[cos(lambdaecliptic);
        cos(E)*sin(lambdaecliptic);
        sin(E)*sin(lambdaecliptic)];  %(m)
  
end

function r = r_moon(T_UT1,Re)

lambdaecliptic = (218.32+481267.8813*T_UT1+6.29*sin((134.9+477198.85*T_UT1)*pi/180)-...
                 1.27*sin((259.2-413335.38*T_UT1)*pi/180)+0.66*sin((235.7+890534.23*T_UT1)*pi/180)+...
                 0.21*sin((269.9+954397.70*T_UT1)*pi/180)-0.19*sin((357.5+35999.05*T_UT1)*pi/180)-...
                 0.11*sin((186.6+966404.05*T_UT1)*pi/180))*pi/180;  %(rad)
phiecliptic = (5.13*sin((93.3+483202.03*T_UT1)*pi/180)+0.28*sin((228.2+960400.87*T_UT1)*pi/180)-...
              0.28*sin((318.3+6003.18*T_UT1)*pi/180)-0.17*sin((217.6-407332.20*T_UT1)*pi/180))*pi/180;  %(rad)
P = (0.9508+0.0518*cos((134.9+477198.85*T_UT1)*pi/180)+0.0095*cos((259.2-413335.38*T_UT1)*pi/180)+...
    0.0078*cos((235.7+890534.23*T_UT1)*pi/180)+0.0028*cos((269.9+954397.70*T_UT1)*pi/180))*pi/180;  %(rad)
epsilon = (23.439291-0.0130042*T_UT1-1.64E-7*T_UT1^2+5.04E-7*T_UT1^3)*pi/180; %rad
radius = Re/sin(P);  %(m)
r = radius*[cos(phiecliptic)*cos(lambdaecliptic);
            cos(epsilon)*cos(phiecliptic)*sin(lambdaecliptic)-sin(epsilon)*sin(phiecliptic);
            sin(epsilon)*cos(phiecliptic)*sin(lambdaecliptic)+cos(epsilon)*sin(phiecliptic)];  %(m)
        
end

function B = Dipole_model(r,GMST,Re)

%2010 IGRF constants
g01 = -29496.5e-9;
g11 = -1585.9e-9;
h11 = 4945.1e-9;

H0 = sqrt(g01^2 + g11^2 + h11^2);

theta_m = acos(g01/H0);
phi_m = atan2(h11,g11);

GMST_m = GMST + phi_m;

m_hat = [sin(theta_m)*cos(GMST_m);
         sin(theta_m)*sin(GMST_m);
         cos(theta_m)];
     
r_hat = r/norm(r);
     
B = Re^3*H0/norm(r)^3*(3*dot(m_hat,r_hat)*r_hat - m_hat);

end

== matlab function ADC_Model/Satellite Dynamics/Spacecraft Plant/MATLAB Function ==
  data: v input; n input; A input; faces input; r input; w_earth input; Re input; A1 output; R_BtoECI input
function A1 = calcArea(v,n,A,faces,r,w_earth,Re,R_BtoECI)
%#codegen

we = [0;0;w_earth];  %spin vector of Earth in ECI frame (rad/s)
v_atmos = cross(we,r);  %velocity of atmosphere (m/s)
v_rel = R_BtoECI'*(v - v_atmos); %velocity of spacecraft relative to atmosphere (m/s)

A1 = 0;
for i =1:faces
    if dot(v_rel/norm(v_rel),n(1:3,i)) > 0
        A1 = A1+dot(v_rel/norm(v_rel),n(1:3,i))*A(i);
    end
end

== matlab function ADC_Model/Satellite Dynamics/Spacecraft Plant/DCM ==
  data: q input; R output
function R = DCM(q)

R = Psi_matrix(q)'*Xi_matrix(q);

end

function A = Xi_matrix(q)
A = [q(4)*eye(3)+skew(q(1:3));
    -q(1:3)'];
end

function A = Psi_matrix(q)
A = [q(4)*eye(3)-skew(q(1:3));
    -q(1:3)'];
end

function A = skew(x)
A = [0 -x(3) x(2);
     x(3) 0  -x(1);
    -x(2) x(1) 0];
end

== matlab function ADC_Model/Satellite Dynamics/Spacecraft Plant/Attitude Dynamics/Plant ==
  data: w_BwrtECI_B input; q_BtoECI_dot output; q_BtoECI input
function q_BtoECI_dot = quat_EOM(w_BwrtECI_B,q_BtoECI)
% This block supports an embeddable subset of the MATLAB language.
% See the help menu for details. 

q_BtoECI_dot = 1/2*Xi_matrix(q_BtoECI)*w_BwrtECI_B;
          
end

function A = Xi_matrix(q)

A = [q(4,1)*eye(3)+skew(q(1:3,1));
    -q(1:3,1)'];
 
end

function A = skew(x)

A = [0    -x(3)  x(2);
     x(3)  0    -x(1);
    -x(2)  x(1)  0];
 
end

== matlab function ADC_Model/Satellite Dynamics/Spacecraft Plant/Disturbances/Aero Drag and Torque/Aerodynamic  Drag and Torque ==
  data: a_aerodrag output; r input; T_aero output; v input; R_BtoECI input; Re input; w_earth input; A input; n input; cp input; faces input; m input
function [a_aerodrag, T_aero] = aero(r,v,R_BtoECI,Re,w_earth,A,n,cp,faces,m)

h = (norm(r) - Re)*10^(-3);  %altitude (km)
we = [0;0;w_earth];  %spin vector of Earth in ECI frame (rad/s)
v_atmos = cross(we,r);  %velocity of atmosphere (m/s)
v_rel = R_BtoECI'*(v - v_atmos); %velocity of spacecraft relative to atmosphere (m/s)

%adding Cd calculations -- KJL 06-03-2013
cmp=sqrt(2*1000*8314/15);
S=norm(v_rel)/cmp;
cmp_w=sqrt(2*300*8314/15);
S_w=norm(v_rel)/cmp_w;
Cd=[0 0 0 0 0 0];

%Scaled height density model
if h < 110
    rho0=5.297e-7;h0=100;SH=5.877;
elseif h >= 110 && h < 120
    rho0=9.661e-8;h0=110;SH=7.263;
elseif h >= 120 && h < 130
    rho0=2.438e-8;h0=120;SH=9.473;
elseif h >= 130 && h < 140
    rho0=8.484e-9;h0=130;SH=12.636;
elseif h >= 140 && h < 150
    rho0=3.845e-9;h0=140;SH=16.149;
elseif h >= 150 && h < 180
    rho0=2.070e-9;h0=150;SH=22.523;
elseif h >= 180 && h < 200
    rho0=5.464e-10;h0=180;SH=29.740;
elseif h >= 200 && h < 250
    rho0=2.789e-10;h0=200;SH=37.105;
elseif h >= 250 && h < 300
    rho0=7.248e-11;h0=250;SH=45.546;
elseif h >= 300 && h < 350
    rho0=2.418e-11;h0=300;SH=53.628;
elseif h >= 350 && h < 400
    rho0=9.518e-12;h0=350;SH=53.298;
elseif h >= 400 && h < 450
    rho0=3.725e-12;h0=400;SH=58.515;
elseif h >= 450 && h < 500
    rho0=1.585e-12;h0=450;SH=60.828;
elseif h >= 500 && h < 600
    rho0=6.967e-13;h0=500;SH=63.822;
elseif h >= 600 && h < 700
    rho0=1.454e-13;h0=600;SH=71.835;
elseif h>= 700 && h < 800
    rho0=3.614e-14;h0=700;SH=88.667;
elseif h >= 800 && h < 900
    rho0=1.170e-14;h0=800;SH=124.64;
elseif h >= 900 && h < 1000
    rho0=5.245e-15;h0=900;SH=181.05;
else%if h > 1000
    rho0=3.019e-15;h0=1000;SH=268.00;
end

rho=rho0*exp(-(h-h0)/SH); %kg/(m^3)

a = [0;0;0];
T = [0;0;0];
for i = 1:faces
    cos_alf = dot(v_rel/norm(v_rel),n(1:3,i));
    alf=acos(cos_alf);
    sin_alf = sin(alf);
    %nsin_alf=-1*sin_alf;
    if cos_alf > 0  %check if face is experiencing drag
        %if cos_alf>0 face is facing ram direction
        Cd(i)=abs(2.2*cos_alf);%(2/(sqrt(pi)*S))*(exp(-(S*sin_alf)^2)+sqrt(pi)*S*sin_alf*(1+1/(2*S^2))*erf(S*sin_alf)+pi*S*sin_alf^2/S_w);
    else %face is in velocity direction
        0;
    end
    a = a + -0.5*Cd(i)/m*rho*A(i)*(v_rel'*v_rel)*v_rel/norm(v_rel);
    F=-0.5*rho*Cd(i)*A(i)*(v_rel'*v_rel)*v_rel/norm(v_rel);
    T = T + cross(cp(1:3,i),F);
end

a_aerodrag = R_BtoECI*a;
T_aero = T;

end

== matlab function ADC_Model/Satellite Dynamics/Spacecraft Plant/Disturbances/Gravity Gradient/Gravity Gradient ==
  data: r input; R_BtoECI input; J_c input; T_GG output; mu input
function T_GG = gravity_gradient(r,R_BtoECI,J_c,mu)

c = R_BtoECI'*r/norm(r); %nadir direction

T_GG = 3*mu/norm(r)^3*cross(c,J_c*c);

end

== matlab function ADC_Model/Satellite Dynamics/Spacecraft Plant/Disturbances/Solar Drag andTorque/Solar Torque ==
  data: a_solardrag output; r input; T_solar output; R_BtoECI input; R_SUN input; Re input; SP input; Cr input; A input; n input; cp input; faces input; m input
function [a_solardrag, T_solar] = solar(r,R_BtoECI,R_SUN,Re,SP,Cr,A,n,cp,faces,m)

temp1 = dot(r/Re,R_SUN/Re);
r1 = norm(r/Re);
r2 = norm(R_SUN/Re);

tau_min = (r1^2 - temp1)/(r1^2 + r2^2 - 2*temp1);

LOS = (tau_min < 0) + (tau_min > 1);
other = (1-tau_min)*r1^2 + temp1*tau_min;
LOS = LOS + (other >= 1);

% rho = asin(Re/(norm(r)));
% Rnadir = -r/norm(r);
% Eclipse = (rho>=acos(dot(Rnadir,R_SUN/norm(R_SUN))));

if LOS
    r_sun = R_BtoECI'*(r-R_SUN);

    a = [0;0;0];
    T = [0;0;0];
    for i = 1:faces
        cos_alf = dot(r_sun/norm(r_sun),n(1:3,i));
        if cos_alf > 0  %check if face is experiencing drag
            a = a + -Cr(i)*SP/m*cos_alf*A(i)*r_sun/norm(r_sun);
            T = T +  Cr(i)*SP*cross(r_sun/norm(r_sun),cp(1:3,i)*cos_alf^2*A(i));
        end
    end
    a_solardrag = R_BtoECI*a;
    T_solar = T;
else
    a_solardrag = [0;0;0];
    T_solar = [0;0;0];
end

end

== matlab function ADC_Model/Satellite Dynamics/Spacecraft Plant/Disturbances/Magnetic Torque/MATLAB Function ==
  data: B input; tauB output; M input
function tauB=Btorque(B,M)
%#codegen

tauB=-skew(B)*M;
end

function A = skew(x)

A = [0    -x(3)  x(2);
     x(3)  0    -x(1);
    -x(2)  x(1)  0];
 
end

== matlab function ADC_Model/Satellite Dynamics/Spacecraft Plant/Disturbances/J2-J6/J2-J6 Effect ==
  data: r_ECI input; R_ECItoECEF input; a_J2to6 output; mu input; Re input; J input
function a_J2to6 = J2to6_pert(r_ECI,R_ECItoECEF,mu,Re,J)

r = R_ECItoECEF*r_ECI;

a_J2 = [-3*J(2)*mu*Re^2*r(1)/(2*(r'*r)^(5/2))*(1-5*r(3)^2/(r'*r));
        -3*J(2)*mu*Re^2*r(2)/(2*(r'*r)^(5/2))*(1-5*r(3)^2/(r'*r));
        -3*J(2)*mu*Re^2*r(3)/(2*(r'*r)^(5/2))*(3-5*r(3)^2/(r'*r))];

a_J3 = [-5*J(3)*mu*Re^3*r(1)/(2*(r'*r)^(7/2))*(3*r(3)-7*r(3)^3/(r'*r));
        -5*J(3)*mu*Re^3*r(2)/(2*(r'*r)^(7/2))*(3*r(3)-7*r(3)^3/(r'*r));
        -5*J(3)*mu*Re^3/(2*(r'*r)^(7/2))*(6*r(3)^2-7*r(3)^4/(r'*r)-3*(r'*r)/5)];

a_J4 = [15*J(4)*mu*Re^4*r(1)/(8*(r'*r)^(7/2))*(1-14*r(3)^2/(r'*r)+21*r(3)^4/(r'*r)^2);
        15*J(4)*mu*Re^4*r(2)/(8*(r'*r)^(7/2))*(1-14*r(3)^2/(r'*r)+21*r(3)^4/(r'*r)^2);
        15*J(4)*mu*Re^4*r(3)/(8*(r'*r)^(7/2))*(5-70*r(3)^2/(3*(r'*r))+21*r(3)^4/(r'*r)^2)];

a_J5 = [3*J(5)*mu*Re^5*r(1)*r(3)/(8*(r'*r)^(9/2))*(35-210*r(3)^2/(r'*r)+231*r(3)^4/(r'*r)^2);
        3*J(5)*mu*Re^5*r(2)*r(3)/(8*(r'*r)^(9/2))*(35-210*r(3)^2/(r'*r)+231*r(3)^4/(r'*r)^2);
        3*J(5)*mu*Re^5*r(3)^2/(8*(r'*r)^(9/2))*(105-315*r(3)^2/(r'*r)+231*r(3)^4/(r'*r)^2)-15*J(5)*mu*Re^5/(8*(r'*r)^(7/2))];

a_J6 = [-J(6)*mu*Re^6*r(1)/(16*(r'*r)^(9/2))*(35-945*r(3)^2/(r'*r)+3465*r(3)^4/(r'*r)^2-3003*r(3)^6/(r'*r)^3);
        -J(6)*mu*Re^6*r(2)/(16*(r'*r)^(9/2))*(35-945*r(3)^2/(r'*r)+3465*r(3)^4/(r'*r)^2-3003*r(3)^6/(r'*r)^3);
        -J(6)*mu*Re^6*r(3)/(16*(r'*r)^(9/2))*(245-2205*r(3)^2/(r'*r)+4851*r(3)^4/(r'*r)^2-3003*r(3)^6/(r'*r)^3)];

a_J2to6 = R_ECItoECEF'*(a_J2 + a_J3 + a_J4 + a_J5 + a_J6);

end

== matlab function ADC_Model/Satellite Dynamics/Spacecraft Plant/Disturbances/3rd Body/Third Body Effects ==
  data: r input; a_3body output; R_SUN input; R_MOON input
function a_3body = third_body_effect(r,R_SUN,R_MOON)

mu_moon = 4902.79882e9;  %gravitational parameter of Moon (m^3/s^2)
mu_sun = 1.32712428e20;  %gravitational parameter of Sun (m^3/s^2)

a_3body = mu_moon*((R_MOON-r)/(norm(R_MOON-r))^3 - R_MOON/(norm(R_MOON))^3) + ...
          mu_sun*((R_SUN-r)/(norm(R_SUN-r))^3 - R_SUN/(norm(R_SUN))^3);

end

== matlab function ADC_Model/Power/Solar_Power/Embedded MATLAB Function ==
  data: Power output; R_SUN input; r input; n input; faces input; Re input; R_BtoECI input; Pfaces input
function Power  = Sun_Power(R_SUN,r,n,faces,Re,R_BtoECI,Pfaces)
efficiency=.25;
AreaPercent=0.95;
SolarIrradiance=1367; % [W/m^2]
r_sun = -R_BtoECI'*(r - R_SUN);

Power = 0;

temp1 = dot(r/Re,R_SUN/Re);
r1 = norm(r/Re);
r2 = norm(R_SUN/Re);
tau_min = (r1^2 - temp1)/(r1^2 + r2^2 - 2*temp1);

LOS = (tau_min < 0) + (tau_min > 1);
other = (1-tau_min)*r1^2 + temp1*tau_min;
LOS = LOS + (other >= 1);

if LOS
    for i = 1:faces
        cos_alf = dot(r_sun/norm(r_sun),n(1:3,i));
        if cos_alf > 0
            Power = Power + cos_alf*Pfaces(i)*efficiency*AreaPercent*SolarIrradiance;
        end
    end
else
    Power = 0;
end
